simulink model "RL"  (Simulink 7.1)
settings: Solver=ode45  StartTime=0.0  StopTime=.02  RelTol=1e-3
undefined symbols (not defined in the file): L, R, V
settings Model: Creator=Smrit  LastModifiedBy=Smrit

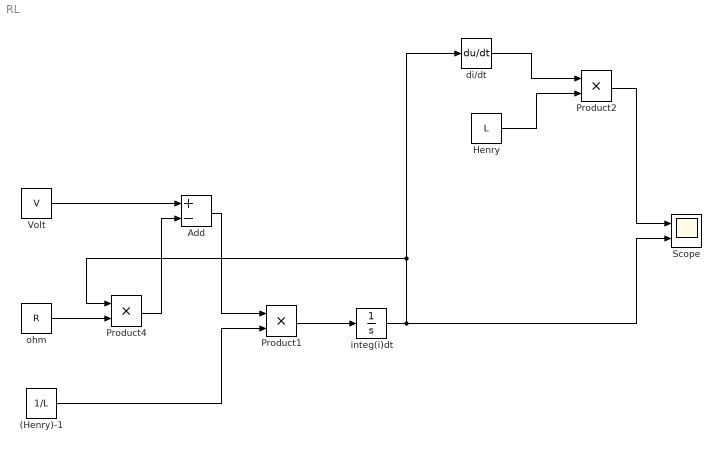
== system RL ==
  (Henry)-1 : Constant  Value=1/L  OutDataType=sfix(16)  OutScaling=2^0
  Add : Sum  Inputs=+-  OutDataType=sfix(16)  OutScaling=2^-10
  Henry : Constant  Value=L  OutDataType=sfix(16)  OutScaling=2^0
  Product1 : Product  OutDataType=sfix(16)  OutScaling=2^0  RndMeth=Zero
  Product2 : Product  OutDataType=sfix(16)  OutScaling=2^0  RndMeth=Zero
  Product4 : Product  OutDataType=sfix(16)  OutScaling=2^0  RndMeth=Zero
  Scope : Scope  NumInputPorts=2
      settings: YMin=-5~-5  YMax=5~5
  Volt : Constant  Value=V  OutDataType=sfix(16)  OutScaling=2^0
  di/dt : Derivative
  integ(i)dt : Integrator
  ohm : Constant  Value=R  OutDataType=sfix(16)  OutScaling=2^0
  wires:
  Volt/1 -> Add/1
  integ(i)dt/1 -> Scope/2, di/dt/1, Product4/1
  ohm/1 -> Product4/2
  (Henry)-1/1 -> Product1/2
  Product1/1 -> integ(i)dt/1
  di/dt/1 -> Product2/1
  Henry/1 -> Product2/2
  Product2/1 -> Scope/1
  Product4/1 -> Add/2
  Add/1 -> Product1/1
